simulink model "HydOilTemp_harness"  (Simulink 7.7)
settings: Solver=FixedStepDiscrete  SolverMode=SingleTasking  StartTime=0.0  StopTime=100  FixedStep=0.1  RelTol=1e-3
InitFcn:
  | CD_HOT_FILTER_GAIN.DataType = 'uint8';
  | CD_HOT_FILTER_GAIN.Value = 3;
  | 
  | if signalbuilder('HydOilTemp_harness/Signal_Builder','activegroup') == 3
  |   CD_SHUTDOWN_FUNCTION.DataType = 'uint8';
  |   CD_SHUTDOWN_FUNCTION.Value = 255;
  | elseif signalbuilder('HydOilTemp_harness/Signal_Builder','activegroup') == 6
  |   CD_SHUTDOWN_FUNCTION.DataType = 'uint8';
  |   CD_SHUTDOWN_FUNCTION.Value = 255;
  | else
  |  CD_SHUTDOWN_FUNCTION.DataType = 'uint8';
  |   CD_SHUTDOWN_FUNCTION.Value = 0;
  | end
  | 
  | if signalbuilder('HydOilTemp_harness/Signal_Builder','activegroup') == 1
  |   CD_HOT_FUNCTION.DataType = 'uint8';
  |   CD_HOT_FUNCTION.Value = 255;
  | elseif signalbuilder('HydOilTemp_harness/Signal_Builder','activegroup') == 5
  |   CD_HOT_FUNCTION.DataType = 'uint8';
  |   CD_HOT_FUNCTION.Value = 1;
  | elseif signalbuilder('HydOilTemp_harness/Signal_Builder','activegroup') == 6
  |   CD_HOT_FUNCTION.DataType = 'uint8';
  |   CD_HOT_FUNCTION.Value = 1;
  | else
  |   CD_HOT_FUNCTION.DataType = 'uint8';
  |   CD_HOT_FUNCTION.Value = 0;
  | end
undefined symbols (not defined in the file): CD_HOT_DEBOUNCE_EXTREMELY_HIGH, CD_HOT_DEBOUNCE_NORMAL, CD_HOT_DEBOUNCE_SHUTDOWN, CD_HOT_SWITCH_EXTREMELY_HIGH, EXTREMELY_HIGH, INIT_NORMAL, MXGTW_HOTGAUGE, MXGTW_HOTSND, NON_FUNCTIONAL, NORMAL, SENDER, SHUTDOWN, sigbuilder_block, srate100, SWITCH_INPUT, SYS_NORMAL
libraries: MX_Library x4, simulink x3
CloseFcn:
  | rtwprivate ssgencode ModelCloseRequest sle_main_controller
settings Model: Creator=smindema  LastModifiedBy=aliebel  RecordCoverage=on  CovMetricSettings=dcmtw  CovHTMLOptions=-aTS=1 -bRG=1 -bTC=1 -hTR=0 -nFC=0 -scm=1 -bcm=1 -xEv=0  CovCumulativeReport=on  CovModelRefEnable=off
settings MATStruct: SampleTime=0.01  Offset=0  Priority=[1.0]
settings DataIOCC: LimitDataPoints=off  SaveOutput=off  SaveTime=off
settings OptimizationCC: BlockReduction=off  InlineParams=on  ExpressionFolding=off  StateBitsets=on  DataBitsets=on  UseTempVars=on  InitFltsAndDblsToZero=on  NoFixptDivByZeroProtection=on  EfficientFloat2IntCast=on  OptimizeModelRefInitCode=on
settings DebuggingCC: SaveWithParameterizedLinksMsg=none  MultiTaskDSMMsg=warning  MultiTaskCondExecSysMsg=none  IntegerOverflowMsg=none  ModelReferenceCSMismatchMessage=warning
settings HardwareCC: ProdBitPerInt=16  ProdBitPerPointer=16  ProdIntDivRoundTo=Floor  ProdEndianess=BigEndian  ProdWordSize=16  ProdHWDeviceType=Motorola HC12
settings ModelReferenceCC: ModelReferenceNumInstancesAllowed=Single
settings RTWCC: SystemTargetFile=ert.tlc  GenCodeOnly=on  TemplateMakefile=ert_default_tmf  Description=Real-Time Workshop Embedded Coder (no auto configuration)  GenerateReport=on  RetainRTWFile=on  ProcessScript=ert_make_rtw_hook  IncludeHyperlinkInReport=on  LaunchReport=on  IncludeERTFirstTime=on
settings RTWCC: CustomHeaderCode=|
  | #include "cpp_req_defines.h"
  | #include "hw_fin.h"
  | #include "cdata.h"
settings CodeAppCC: IgnoreCustomStorageClasses=off  DefineNamingRule=UpperCase
settings ERTTargetCC: TargetFcnLib=ansi_tfl_tmw.mat  FunctionExecutionProfile=off  MultiwordLength=2048  GenerateSampleERTMain=on  IncludeMdlTerminateFcn=off  SupportAbsoluteTime=off  SupportNonFinite=off  SupportComplex=off  PurelyIntegerCode=on  ERTCustomFileTemplate=gen_rtw_req_defines_h.tlc  GlobalDataDefinition=InSeparateSourceFile  GlobalDataReference=InSeparateHeaderFile  ConvertIfToSwitch=off

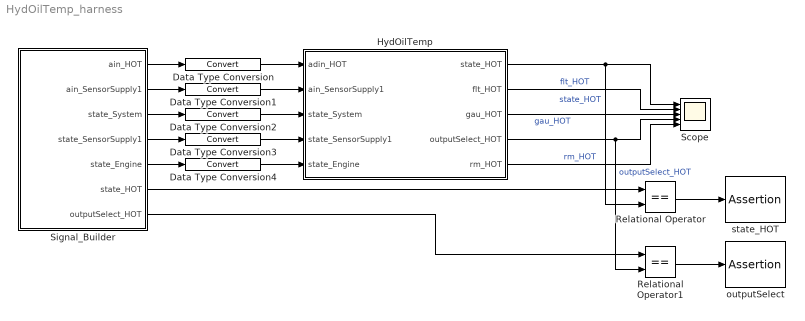
== system HydOilTemp_harness ==
  Data Type Conversion{,1..4} (5 alike) : DataTypeConversion
  HydOilTemp : Subsystem  TreatAsAtomicUnit=on  SystemSampleTime=srate100  RTWFileName=mod_Inputs
      settings: RTWSystemCode=Function  RTWFcnNameOpts=Use subsystem name  RTWFileNameOpts=User specified
  Relational Operator : RelationalOperator  Operator===  OutDataTypeStr=boolean
  Relational Operator1 : RelationalOperator  Operator===  OutDataTypeStr=boolean
  Scope : Scope  NumInputPorts=5
      settings: TimeRange=100  YMin=8~125~0~-1~550  YMax=15~350~17.5~1~950  MaxDataPoints=50000
  Signal_Builder : Subsystem  Tag=STV Subsys  LoadFcn=sigbuilder_block('load');  StartFcn=sigbuilder_block('start');  StopFcn=sigbuilder_block('stop');  ClipboardFcn=sigbuilder_block('clipboard');  mask(Sigbuilder block){}
      mask help: Sigbuilder GUI
      mask init:
      | if ~strcmp(get_param(bdroot(gcbh),'SimulationStatus'),'stopped') tuvar = sigbuilder_block('maskInit'); end
      settings: CopyFcn=sigbuilder_block('copy');  DeleteFcn=sigbuilder_block('delete');  ModelCloseFcn=sigbuilder_block('modelClose');  PreSaveFcn=sigbuilder_block('preSave');  NameChangeFcn=sigbuilder_block('namechange');  OpenFcn=sigbuilder_block('open',[348 297.75 957.75 420.75 ]);  CloseFcn=sigbuilder_block('close');
      mask Display: plot(0,0,100,100,[10,10,40,40,10],[80,20,20,80,80],[40,10],[50,50], [40,27,10],[65,72,56],[40,25,25,10],[28,28,43,43]);
  outputSelect : Assertion  Enabled=off
  state_HOT : Assertion  Enabled=off
  wires:
  Signal_Builder/1(ain_HOT) -> Data Type Conversion/1
  Signal_Builder/2(ain_SensorSupply1) -> Data Type Conversion1/1
  Data Type Conversion/1 -> HydOilTemp/1(adin_HOT)
  HydOilTemp/1(state_HOT) -> Scope/1, Relational Operator/2  "state_HOT"
  HydOilTemp/2(flt_HOT) -> Scope/2  "flt_HOT"
  HydOilTemp/3(gau_HOT) -> Scope/3  "gau_HOT"
  HydOilTemp/4(outputSelect_HOT) -> Scope/4, Relational Operator1/2  "outputSelect_HOT"
  HydOilTemp/5(rm_HOT) -> Scope/5  "rm_HOT"
  Data Type Conversion1/1 -> HydOilTemp/2(ain_SensorSupply1)
  Data Type Conversion2/1 -> HydOilTemp/3(state_System)
  Data Type Conversion3/1 -> HydOilTemp/4(state_SensorSupply1)
  Data Type Conversion4/1 -> HydOilTemp/5(state_Engine)
  Signal_Builder/3(state_System) -> Data Type Conversion2/1
  Signal_Builder/4(state_SensorSupply1) -> Data Type Conversion3/1
  Signal_Builder/5(state_Engine) -> Data Type Conversion4/1
  Relational Operator/1 -> state_HOT/1
  Relational Operator1/1 -> outputSelect/1
  Signal_Builder/6(state_HOT) -> Relational Operator/1
  Signal_Builder/7(outputSelect_HOT) -> Relational Operator1/1

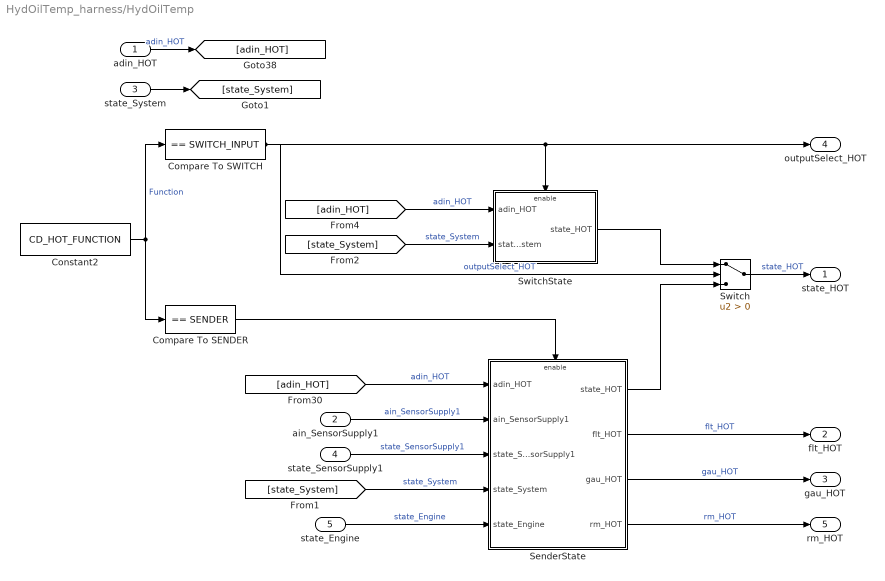
== system HydOilTemp_harness/HydOilTemp ==
  adin_HOT : Inport  OutDataTypeStr=uint16
  ain_SensorSupply1 : Inport  Port=2  OutDataTypeStr=uint16
  state_System : Inport  Port=3
  state_SensorSupply1 : Inport  Port=4  OutDataTypeStr=uint8
  state_Engine : Inport  Port=5  OutDataTypeStr=uint8
  Compare To SENDER : simulink/Logic and Bit Operations/Compare To Constant  SystemSampleTime=-1  relop===  const=SENDER  LogicOutDataTypeMode=boolean  ZeroCross=off
  Compare To SWITCH : simulink/Logic and Bit Operations/Compare To Constant  SystemSampleTime=-1  relop===  const=SWITCH_INPUT  LogicOutDataTypeMode=boolean  ZeroCross=off
  Constant2 : Constant  Value=CD_HOT_FUNCTION  OutDataTypeStr=uint8
  SenderState : Subsystem  TreatAsAtomicUnit=on
  Switch : Switch  Criteria=u2 > Threshold  ZeroCross=off
      settings: AttributesFormatString=<threshold=%<Threshold>>
  SwitchState : Subsystem  TreatAsAtomicUnit=on
  state_HOT : Outport  OutDataTypeStr=uint8
  flt_HOT : Outport  Port=2  OutDataTypeStr=uint16
  gau_HOT : Outport  Port=3  OutDataTypeStr=uint16
  outputSelect_HOT : Outport  Port=4
  rm_HOT : Outport  Port=5  OutDataTypeStr=uint16
  wires:
  state_SensorSupply1/1 -> SenderState/3(state_SensorSupply1)  "state_SensorSupply1"
  ain_SensorSupply1/1 -> SenderState/2(ain_SensorSupply1)  "ain_SensorSupply1"
  [adin_HOT] -> SenderState/1(adin_HOT)  "adin_HOT"
  [adin_HOT] -> SwitchState/1(adin_HOT)  "adin_HOT"
  Switch/1 -> state_HOT/1  "state_HOT"
  SwitchState/1(state_HOT) -> Switch/1
  SenderState/1(state_HOT) -> Switch/3
  SenderState/3(gau_HOT) -> gau_HOT/1  "gau_HOT"
  SenderState/2(flt_HOT) -> flt_HOT/1  "flt_HOT"
  adin_HOT/1 -> [adin_HOT]  "adin_HOT"
  Constant2/1 -> Compare To SWITCH/1, Compare To SENDER/1  "Function"
  Compare To SENDER/1 -> SenderState/Enable
  Compare To SWITCH/1 -> Switch/2, SwitchState/Enable, outputSelect_HOT/1  "outputSelect_HOT"
  [state_System] -> SenderState/4(state_System)  "state_System"
  state_System/1 -> [state_System]
  [state_System] -> SwitchState/2(state_System)  "state_System"
  SenderState/4(rm_HOT) -> rm_HOT/1  "rm_HOT"
  state_Engine/1 -> SenderState/5(state_Engine)  "state_Engine"

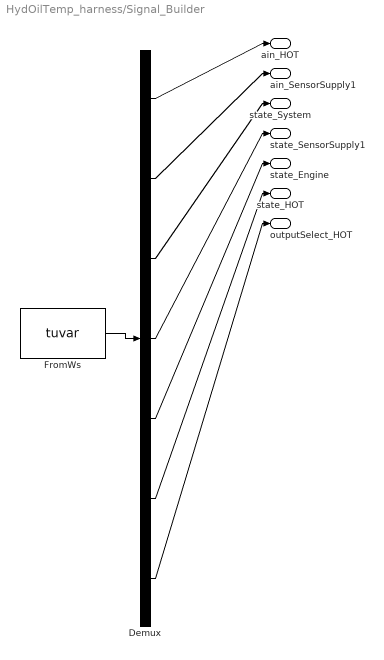
== system HydOilTemp_harness/Signal_Builder ==
  Demux : Demux  Tag=STV Demux  Outputs=7
  FromWs : FromWorkspace  Tag=STV FromWs  VariableName=tuvar  SampleTime=0  SigBuilderData=DataTag0  VnvData=DataTag1
      SigBuilderData=|
      | common.afterFinalStr = 'Extrapolate'
      | common.sampleTime = 0
      | dataSet(1).timeRange = [0 100]
      | dataSet(1).name = 'T1-Nonfunc'
      | dataSet(2).timeRange = [0 100]
      | dataSet(2).name = 'T2-OOR'
      | dataSet(3).timeRange = [0 100]
      | dataSet(3).name = 'T3-HIGH'
      | dataSet(4).timeRange = [0 100]
      | dataSet(4).name = 'T4-EXTHIGH'
      | dataSet(5).timeRange = [0 100]
      | dataSet(5).name = 'T5-SWITCH'
      | dataSet(6).timeRange = [0 100]
      | dataSet(6).name = 'T6-SWITCH no shut'
      | dataSet(7).timeRange = [0 100]
      | dataSet(7).name = 'TABLE'
      | dataSet(8).timeRange = [0 100]
      | dataSet(8).name = 'TABLE1'
      | sbobj.Groups(1).Name = 'T1-Nonfunc'
      | sbobj.Groups(1).Signals(1).Name = 'ain_HOT'
      | sbobj.Groups(1).Signals(1).XData = [0 100]
      | sbobj.Groups(1).Signals(1).YData = [380 380]
      | sbobj.Groups(1).Signals(2).Name = 'ain_SensorSupply1'
      | sbobj.Groups(1).Signals(2).XData = [0 100]
      | sbobj.Groups(1).Signals(2).YData = [850 850]
      | sbobj.Groups(1).Signals(3).Name = 'state_System'
      | sbobj.Groups(1).Signals(3).XData = [0 0.6 0.6 100]
      | sbobj.Groups(1).Signals(3).YData = [0 0 1 1]
      | sbobj.Groups(1).Signals(4).Name = 'state_SensorSupply1'
      | sbobj.Groups(1).Signals(4).XData = [0 100]
      | sbobj.Groups(1).Signals(4).YData = [8 8]
      | sbobj.Groups(1).Signals(5).Name = 'state_Engine'
      | sbobj.Groups(1).Signals(5).XData = [0 100]
      | sbobj.Groups(1).Signals(5).YData = [3 3]
      | sbobj.Groups(1).Signals(6).Name = 'state_HOT'
      | sbobj.Groups(1).Signals(6).XData = [0 100]
      | sbobj.Groups(1).Signals(6).YData = [8 8]
      | sbobj.Groups(1).Signals(7).Name = 'outputSelect_HOT'
      | sbobj.Groups(1).Signals(7).XData = [0 100]
      | sbobj.Groups(1).Signals(7).YData = [0 0]
      | sbobj.Groups(2).Name = 'T2-OOR'
      | sbobj.Groups(2).Signals(1).Name = 'ain_HOT'
      | sbobj.Groups(2).Signals(1).XData = [0 0.4 0.4 0.9 0.9 34.6 34.6 35 35 36.3 36.3 38.4 38.4 39.7 39.7 40.4 40.4 75 75 75.4 75.4 76.3 76.3 100]
      | sbobj.Groups(2).Signals(1).YData = [0 0 600 600 0 0 280 290 0 0 500 500 1020 1010 420 430 1020 1020 230 240 1000 998.269230769 640 640]
      | sbobj.Groups(2).Signals(2).Name = 'ain_SensorSupply1'
      | sbobj.Groups(2).Signals(2).XData = [0 100]
      | sbobj.Groups(2).Signals(2).YData = [850 850]
      | sbobj.Groups(2).Signals(3).Name = 'state_System'
      | sbobj.Groups(2).Signals(3).XData = [0 0.2 0.2 100]
      | sbobj.Groups(2).Signals(3).YData = [0 0 1 1]
      | sbobj.Groups(2).Signals(4).Name = 'state_SensorSupply1'
      | sbobj.Groups(2).Signals(4).XData = [0 2.7 2.7 3.1 3.1 33.6 33.6 33.8 33.8 41.8 41.8 42.4 42.4 73.1 73.1 73.8 73.8 100]
      | sbobj.Groups(2).Signals(4).YData = [8 8 6.98 6.98 8 8 6.98 6.98 8 8 7 7 8 8 7 7 8 8]
      | sbobj.Groups(2).Signals(5).Name = 'state_Engine'
      | sbobj.Groups(2).Signals(5).XData = [0 100]
      | sbobj.Groups(2).Signals(5).YData = [0 0]
      | sbobj.Groups(2).Signals(6).Name = 'state_HOT'
      | sbobj.Groups(2).Signals(6).XData = [0 33.3 33.3 41.8 41.8 72.6 72.6 81.4 81.4 100]
      | sbobj.Groups(2).Signals(6).YData = [8 8 22 22 8 8 21 21 8 8]
      | sbobj.Groups(2).Signals(7).Name = 'outputSelect_HOT'
      | sbobj.Groups(2).Signals(7).XData = [0 100]
      | sbobj.Groups(2).Signals(7).YData = [0 0]
      | sbobj.Groups(3).Name = 'T3-HIGH'
      | sbobj.Groups(3).Signals(1).Name = 'ain_HOT'
      | sbobj.Groups(3).Signals(1).XData = [0 2.2 2.2 7 7 7.5 7.5 18.2 18.2 18.5 18.5 29.7 29.7 30.8 30.8 31.7 31.7 39 39 39.5 39.5 50.1 50.1 55.4 55.4 63.6 63.6 64.1 64.1 70.1 70.1 76.4 76.4 77.6 77.6 83.8 83.8 94.8 94.8 97.8 97.8 100]
      | sbobj.Groups(3).Signals(1).YData = [500 500 695 695 500 495 695 695 500 500 695 695 455 450 600 600 455 455 600 600 455 455 700 700 780 780 635 635 780 780 700 700 600 600 700 700 590 590 770 770 590 590]
      | sbobj.Groups(3).Signals(2).Name = 'ain_SensorSupply1'
      | sbobj.Groups(3).Signals(2).XData = [0 100]
      | sbobj.Groups(3).Signals(2).YData = [850 850]
      | sbobj.Groups(3).Signals(3).Name = 'state_System'
      | sbobj.Groups(3).Signals(3).XData = [0 100]
      | sbobj.Groups(3).Signals(3).YData = [1 1]
      | sbobj.Groups(3).Signals(4).Name = 'state_SensorSupply1'
      | sbobj.Groups(3).Signals(4).XData = [0 100]
      | sbobj.Groups(3).Signals(4).YData = [8 8]
      | sbobj.Groups(3).Signals(5).Name = 'state_Engine'
      | sbobj.Groups(3).Signals(5).XData = [0 3.7 3.7 22.8 22.8 24.3 24.3 41.7 41.7 42.3 42.3 67 67 67.9 67.9 100]
      | sbobj.Groups(3).Signals(5).YData = [0 0 3 3 1 1 3 3 1 1 3 3 0.95 0.95 3 3]
      | sbobj.Groups(3).Signals(6).Name = 'state_HOT'
      | sbobj.Groups(3).Signals(6).XData = [0 14.7 14.7 37 37 63.4 63.4 89 89 100]
      | sbobj.Groups(3).Signals(6).YData = [8 8 10 10 12 12 11 11 8 8]
      | sbobj.Groups(3).Signals(7).Name = 'outputSelect_HOT'
      | sbobj.Groups(3).Signals(7).XData = [0 100]
      | sbobj.Groups(3).Signals(7).YData = [0 0]
      | sbobj.Groups(4).Name = 'T4-EXTHIGH'
      | sbobj.Groups(4).Signals(1).Name = 'ain_HOT'
      | sbobj.Groups(4).Signals(1).XData = [0 1 1 8.9 8.9 21 21 21.4 21.4 58.4 58.4 76.4 76.4 77.6 77.6 83.8 83.8 94.8 94.8 97.8 97.8 100]
      | sbobj.Groups(4).Signals(1).YData = [1040 1040 700 700 770 770 400 400 770 780 700 700 600 600 700 700 590 590 770 770 590 590]
      | sbobj.Groups(4).Signals(2).Name = 'ain_SensorSupply1'
      | sbobj.Groups(4).Signals(2).XData = [0 87.2 100]
      | sbobj.Groups(4).Signals(2).YData = [850 850 850]
      | sbobj.Groups(4).Signals(3).Name = 'state_System'
      | sbobj.Groups(4).Signals(3).XData = [0 0.7 0.7 91.9 91.9 93 93 100]
      | sbobj.Groups(4).Signals(3).YData = [0 0 1 1 0 0 1 1]
      | sbobj.Groups(4).Signals(4).Name = 'state_SensorSupply1'
      | sbobj.Groups(4).Signals(4).XData = [0 85 85 87 87 100]
      | sbobj.Groups(4).Signals(4).YData = [8 8 7 7 8 8]
      | sbobj.Groups(4).Signals(5).Name = 'state_Engine'
      | sbobj.Groups(4).Signals(5).XData = [0 32 32 33.7 33.7 100]
      | sbobj.Groups(4).Signals(5).YData = [3 3 2 2 3 3]
      | sbobj.Groups(4).Signals(6).Name = 'state_HOT'
      | sbobj.Groups(4).Signals(6).XData = [0 15 15 54 54 85 85 100]
      | sbobj.Groups(4).Signals(6).YData = [8 8 11 11 15 15 8 8]
      | sbobj.Groups(4).Signals(7).Name = 'outputSelect_HOT'
      | sbobj.Groups(4).Signals(7).XData = [0 100]
      | sbobj.Groups(4).Signals(7).YData = [0 0]
      | sbobj.Groups(5).Name = 'T5-SWITCH'
      | sbobj.Groups(5).Signals(1).Name = 'ain_HOT'
      | sbobj.Groups(5).Signals(1).XData = [0 9.8 9.8 13 13 18 18 20 20 22 22 34 34 35.4 35.4 50 50 60.8 60.8 97.8 97.8 100]
      | sbobj.Groups(5).Signals(1).YData = [1024 1024 0 0 1024 1024 0 0 1000 1000 0 0 980 980 0 0 1024 1024 0 0 1040 1040]
      | sbobj.Groups(5).Signals(2).Name = 'ain_SensorSupply1'
      | sbobj.Groups(5).Signals(2).XData = [0 100]
      | sbobj.Groups(5).Signals(2).YData = [850 850]
      | sbobj.Groups(5).Signals(3).Name = 'state_System'
      | sbobj.Groups(5).Signals(3).XData = [0 8.6 8.6 11.5 11.5 100]
      | sbobj.Groups(5).Signals(3).YData = [1 1 0 0 1 1]
      | sbobj.Groups(5).Signals(4).Name = 'state_SensorSupply1'
      | sbobj.Groups(5).Signals(4).XData = [0 100]
      | sbobj.Groups(5).Signals(4).YData = [8 8]
      | sbobj.Groups(5).Signals(5).Name = 'state_Engine'
      | sbobj.Groups(5).Signals(5).XData = [0 100]
      | sbobj.Groups(5).Signals(5).YData = [0 0]
      | sbobj.Groups(5).Signals(6).Name = 'state_HOT'
      | sbobj.Groups(5).Signals(6).XData = [0 32.1 32.1 55.2 55.2 70.9 70.9 91.1 91.1 100]
      | sbobj.Groups(5).Signals(6).YData = [8 8 11 11 8 8 11 11 15 15]
      | sbobj.Groups(5).Signals(7).Name = 'outputSelect_HOT'
      | sbobj.Groups(5).Signals(7).XData = [0 100]
      | sbobj.Groups(5).Signals(7).YData = [1 1]
      | sbobj.Groups(6).Name = 'T6-SWITCH no shut'
      | sbobj.Groups(6).Signals(1).Name = 'ain_HOT'
      | sbobj.Groups(6).Signals(1).XData = [0 9.8 9.8 13 13 18 18 20 20 22 22 42.6 42.6 44.8 44.8 50 50 60.8 60.8 79.4 79.4 100]
      | sbobj.Groups(6).Signals(1).YData = [1024 1024 0 0 1024 1024 0 0 1000 1000 0 0 980 980 0 0 1024 1024 0 0 1040 1040]
      | sbobj.Groups(6).Signals(2).Name = 'ain_SensorSupply1'
      | sbobj.Groups(6).Signals(2).XData = [0 100]
      | sbobj.Groups(6).Signals(2).YData = [850 850]
      | sbobj.Groups(6).Signals(3).Name = 'state_System'
      | sbobj.Groups(6).Signals(3).XData = [0 8.6 8.6 11.5 11.5 28.2 28.2 31 31 72.1 72.1 82.8 82.8 100]
      | sbobj.Groups(6).Signals(3).YData = [1 1 0 0 1 1 0 0 1 1 0 0 1 1]
      | sbobj.Groups(6).Signals(4).Name = 'state_SensorSupply1'
      | sbobj.Groups(6).Signals(4).XData = [0 100]
      | sbobj.Groups(6).Signals(4).YData = [8 8]
      | sbobj.Groups(6).Signals(5).Name = 'state_Engine'
      | sbobj.Groups(6).Signals(5).XData = [0 100]
      | sbobj.Groups(6).Signals(5).YData = [0 0]
      | sbobj.Groups(6).Signals(6).Name = 'state_HOT'
      | sbobj.Groups(6).Signals(6).XData = [0 41.1 41.1 55.1 55.1 70.9 70.9 77.2 77.2 100]
      | sbobj.Groups(6).Signals(6).YData = [8 8 11 11 8 8 11 11 8 8]
      | sbobj.Groups(6).Signals(7).Name = 'outputSelect_HOT'
      | sbobj.Groups(6).Signals(7).XData = [0 100]
      | sbobj.Groups(6).Signals(7).YData = [1 1]
      | sbobj.Groups(7).Name = 'TABLE'
      | sbobj.Groups(7).Signals(1).Name = 'ain_HOT'
      | sbobj.Groups(7).Signals(1).XData = [0 100]
      | sbobj.Groups(7).Signals(1).YData = [500 1024]
      | sbobj.Groups(7).Signals(2).Name = 'ain_SensorSupply1'
      | sbobj.Groups(7).Signals(2).XData = [0 100]
      | sbobj.Groups(7).Signals(2).YData = [850 850]
      | sbobj.Groups(7).Signals(3).Name = 'state_System'
      | sbobj.Groups(7).Signals(3).XData = [0 0.6 0.6 100]
      | sbobj.Groups(7).Signals(3).YData = [0 0 1 1]
      | sbobj.Groups(7).Signals(4).Name = 'state_SensorSupply1'
      | sbobj.Groups(7).Signals(4).XData = [0 100]
      | sbobj.Groups(7).Signals(4).YData = [8 8]
      | sbobj.Groups(7).Signals(5).Name = 'state_Engine'
      | sbobj.Groups(7).Signals(5).XData = [0 100]
      | sbobj.Groups(7).Signals(5).YData = [3 3]
      | sbobj.Groups(7).Signals(6).Name = 'state_HOT'
      | sbobj.Groups(7).Signals(6).XData = [0 5.8 5.8 15.6 15.6 48.4 48.4 84.8 84.8 100]
      | sbobj.Groups(7).Signals(6).YData = [8 8 12 12 8 8 11 11 21 21]
      | sbobj.Groups(7).Signals(7).Name = 'outputSelect_HOT'
      | sbobj.Groups(7).Signals(7).XData = [0 100]
      | sbobj.Groups(7).Signals(7).YData = [0 0]
      | sbobj.Groups(8).Name = 'TABLE1'
      | sbobj.Groups(8).Signals(1).Name = 'ain_HOT'
      | sbobj.Groups(8).Signals(1).XData = [0 100]
      | sbobj.Groups(8).Signals(1).YData = [500 0]
      | sbobj.Groups(8).Signals(2).Name = 'ain_SensorSupply1'
      | sbobj.Groups(8).Signals(2).XData = [0 100]
      | sbobj.Groups(8).Signals(2).YData = [850 850]
      | sbobj.Groups(8).Signals(3).Name = 'state_System'
      | sbobj.Groups(8).Signals(3).XData = [0 0.6 0.6 100]
      | sbobj.Groups(8).Signals(3).YData = [0 0 1 1]
      | sbobj.Groups(8).Signals(4).Name = 'state_SensorSupply1'
      | sbobj.Groups(8).Signals(4).XData = [0 100]
      | sbobj.Groups(8).Signals(4).YData = [8 8]
      | sbobj.Groups(8).Signals(5).Name = 'state_Engine'
      | sbobj.Groups(8).Signals(5).XData = [0 100]
      | sbobj.Groups(8).Signals(5).YData = [3 3]
      | sbobj.Groups(8).Signals(6).Name = 'state_HOT'
      | sbobj.Groups(8).Signals(6).XData = [0 5.8 5.8 100]
      | sbobj.Groups(8).Signals(6).YData = [8 8 12 12]
      | sbobj.Groups(8).Signals(7).Name = 'outputSelect_HOT'
      | sbobj.Groups(8).Signals(7).XData = [0 100]
      | sbobj.Groups(8).Signals(7).YData = [0 0]
  ain_HOT : Outport  Tag=STV Outport
  ain_SensorSupply1 : Outport  Tag=STV Outport  Port=2
  state_System : Outport  Tag=STV Outport  Port=3
  state_SensorSupply1 : Outport  Tag=STV Outport  Port=4
  state_Engine : Outport  Tag=STV Outport  Port=5
  state_HOT : Outport  Tag=STV Outport  Port=6
  outputSelect_HOT : Outport  Tag=STV Outport  Port=7
  wires:
  FromWs/1 -> Demux/1
  Demux/1 -> ain_HOT/1
  Demux/2 -> ain_SensorSupply1/1
  Demux/3 -> state_System/1
  Demux/4 -> state_SensorSupply1/1
  Demux/5 -> state_Engine/1
  Demux/6 -> state_HOT/1
  Demux/7 -> outputSelect_HOT/1

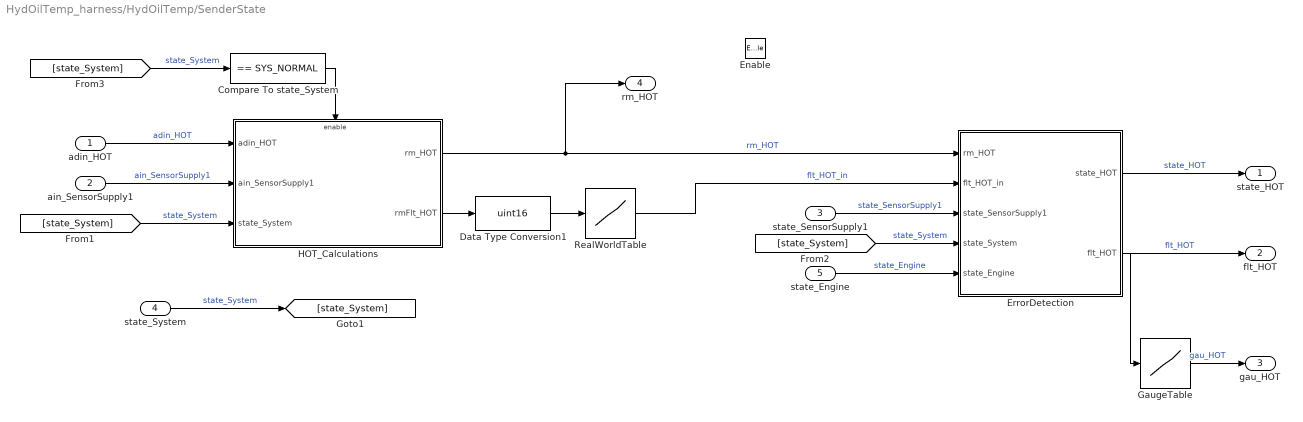
== system HydOilTemp_harness/HydOilTemp/SenderState ==
  adin_HOT : Inport  OutDataTypeStr=uint16
  ain_SensorSupply1 : Inport  Port=2  OutDataTypeStr=uint16
  state_SensorSupply1 : Inport  Port=3  OutDataTypeStr=uint8
  state_System : Inport  Port=4
  state_Engine : Inport  Port=5
  Enable : EnablePort  PropagateVarSize=During execution
      settings: AttributesFormatString=<state=%<StatesWhenEnabling>>
  Compare To state_System : simulink/Logic and Bit Operations/Compare To Constant  SystemSampleTime=-1  relop===  const=SYS_NORMAL  LogicOutDataTypeMode=boolean  ZeroCross=off
  Data Type Conversion1 : DataTypeConversion  OutDataTypeStr=uint16
  ErrorDetection : Stateflow chart  TreatAsAtomicUnit=on
  GaugeTable : Lookup  InputValues=[0:340]  Table=MXGTW_HOTGAUGE  LookUpMeth=Use Input Nearest  OutDataTypeStr=uint16  RndMeth=Zero  SaturateOnIntegerOverflow=on
      settings: AttributesFormatString=input = %<InputValues>\noutput = %<OutputValues>\nlookup = %<LookUpMeth>\nrounding = %<RndMeth>
  HOT_Calculations : Subsystem
  RealWorldTable : Lookup  InputValues=MXGTW_HOTSND  Table=[0:340]  LookUpMeth=Use Input Nearest  OutDataTypeStr=uint16  RndMeth=Zero  SaturateOnIntegerOverflow=on
      settings: AttributesFormatString=input = %<InputValues>\noutput = %<OutputValues>\nlookup = %<LookUpMeth>\nrounding = %<RndMeth>
  state_HOT : Outport  InitialOutput=[INIT_NORMAL]
  flt_HOT : Outport  Port=2  InitialOutput=[0]
  gau_HOT : Outport  Port=3  InitialOutput=[0]
  rm_HOT : Outport  Port=4  InitialOutput=[0]
  wires:
  state_SensorSupply1/1 -> ErrorDetection/3(state_SensorSupply1)  "state_SensorSupply1"
  ErrorDetection/1(state_HOT) -> state_HOT/1  "state_HOT"
  GaugeTable/1 -> gau_HOT/1  "gau_HOT"
  RealWorldTable/1 -> ErrorDetection/2(flt_HOT_in)  "flt_HOT_in"
  ain_SensorSupply1/1 -> HOT_Calculations/2(ain_SensorSupply1)  "ain_SensorSupply1"
  adin_HOT/1 -> HOT_Calculations/1(adin_HOT)  "adin_HOT"
  HOT_Calculations/2(rmFlt_HOT) -> Data Type Conversion1/1
  [state_System] -> ErrorDetection/4(state_System)  "state_System"
  state_Engine/1 -> ErrorDetection/5(state_Engine)  "state_Engine"
  ErrorDetection/2(flt_HOT) -> flt_HOT/1, GaugeTable/1  "flt_HOT"
  state_System/1 -> [state_System]  "state_System"
  HOT_Calculations/1(rm_HOT) -> ErrorDetection/1(rm_HOT), rm_HOT/1  "rm_HOT"
  [state_System] -> HOT_Calculations/3(state_System)  "state_System"
  Data Type Conversion1/1 -> RealWorldTable/1
  Compare To state_System/1 -> HOT_Calculations/Enable
  [state_System] -> Compare To state_System/1  "state_System"

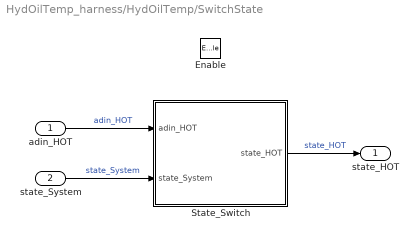
== system HydOilTemp_harness/HydOilTemp/SwitchState ==
  adin_HOT : Inport
  state_System : Inport  Port=2
  Enable : EnablePort  PropagateVarSize=During execution
      settings: AttributesFormatString=<state=%<StatesWhenEnabling>>
  State_Switch : Stateflow chart  TreatAsAtomicUnit=on
  state_HOT : Outport  InitialOutput=[INIT_NORMAL]
  wires:
  State_Switch/1(state_HOT) -> state_HOT/1  "state_HOT"
  adin_HOT/1 -> State_Switch/1(adin_HOT)  "adin_HOT"
  state_System/1 -> State_Switch/2(state_System)  "state_System"

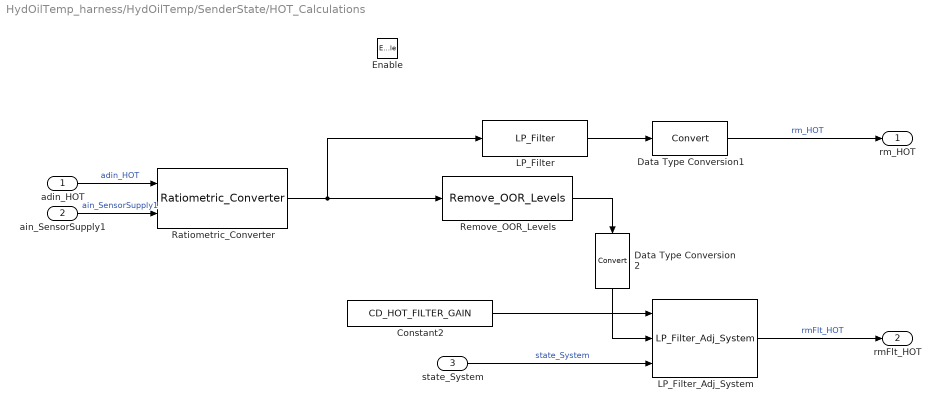
== system HydOilTemp_harness/HydOilTemp/SenderState/HOT_Calculations ==
  adin_HOT : Inport  OutDataTypeStr=uint16
  ain_SensorSupply1 : Inport  Port=2  OutDataTypeStr=uint16
  state_System : Inport  Port=3  OutDataTypeStr=uint8
  Enable : EnablePort  StatesWhenEnabling=reset  PropagateVarSize=During execution
  Constant2 : Constant  Value=CD_HOT_FILTER_GAIN  OutDataTypeStr=uint8
  Data Type Conversion1 : DataTypeConversion
  Data Type Conversion2 : DataTypeConversion
  LP_Filter : MX_Library/LP_Filter  SystemSampleTime=-1  GAIN=3
  LP_Filter_Adj_System : MX_Library/LP_Filter_Adj_System  SystemSampleTime=-1
  Ratiometric_Converter : MX_Library/Ratiometric_Converter  SystemSampleTime=-1  multiplier=1000
  Remove_OOR_Levels : MX_Library/Remove_OOR_Levels  SystemSampleTime=-1  OORL_LEVEL=CD_HOT_OORL  OORH_LEVEL=CD_HOT_OORH
  rm_HOT : Outport  InitialOutput=[0]
  rmFlt_HOT : Outport  Port=2  InitialOutput=[0]
  wires:
  Remove_OOR_Levels/1 -> Data Type Conversion2/1
  Data Type Conversion1/1 -> rm_HOT/1  "rm_HOT"
  Ratiometric_Converter/1 -> Remove_OOR_Levels/1, LP_Filter/1
  ain_SensorSupply1/1 -> Ratiometric_Converter/2  "ain_SensorSupply1"
  adin_HOT/1 -> Ratiometric_Converter/1  "adin_HOT"
  LP_Filter_Adj_System/1 -> rmFlt_HOT/1  "rmFlt_HOT"
  Data Type Conversion2/1 -> LP_Filter_Adj_System/2
  LP_Filter/1 -> Data Type Conversion1/1
  Constant2/1 -> LP_Filter_Adj_System/1
  state_System/1 -> LP_Filter_Adj_System/3  "state_System"

== stateflow chart HydOilTemp/SwitchState/State_Switch ==
  state NORMAL
    state NORMAL
      en:state_HOT = NORMAL;
    state DEBOUNCE
      en:debounceCount = 0;
      du:debounceCount++;
    (default) -> NORMAL.DEBOUNCE
    NORMAL.DEBOUNCE -> NORMAL.NORMAL : [(debounceCount >= CD_HOT_DEBOUNCE_NORMAL)...
        | || (state_HOT == NORMAL)]
  state SHUTDOWN
    state DEBOUNCE
      en:debounceCount = 0;
      du:debounceCount++;
    state SHUTDOWN
      en:state_HOT = SHUTDOWN;
    (default) -> SHUTDOWN.DEBOUNCE
    SHUTDOWN.DEBOUNCE -> SHUTDOWN.SHUTDOWN : [(debounceCount >= CD_HOT_DEBOUNCE_SHUTDOWN)]
  state EXTREMELY_HIGH
    state EXTREMELY_HIGH
      en:state_HOT = EXTREMELY_HIGH;
    state DEBOUNCE
      en:debounceCount = 0;
      du:debounceCount++;
    EXTREMELY_HIGH.DEBOUNCE -> EXTREMELY_HIGH.EXTREMELY_HIGH : [(debounceCount >= CD_HOT_DEBOUNCE_EXTREMELY_HIGH)...
        | || (state_HOT== EXTREMELY_HIGH)]
    (default) -> EXTREMELY_HIGH.DEBOUNCE
  NORMAL -> EXTREMELY_HIGH : [(adin_HOT <= CD_HOT_SWITCH_EXTREMELY_HIGH)...
      | && (state_System == SYS_NORMAL)]
  SHUTDOWN -> EXTREMELY_HIGH : [(adin_HOT > CD_HOT_SWITCH_EXTREMELY_HIGH)...
      | && (state_HOT != SHUTDOWN)]
  EXTREMELY_HIGH -> NORMAL [order 1] : [(adin_HOT > CD_HOT_SWITCH_EXTREMELY_HIGH)...
      | || (state_System != SYS_NORMAL)]
  EXTREMELY_HIGH -> SHUTDOWN [order 2] : [(CD_SHUTDOWN_FUNCTION != NON_FUNCTIONAL)...
      | && (state_HOT == EXTREMELY_HIGH)]
  (default) -> NORMAL.NORMAL
  data: adin_HOT input uint16; state_HOT output uint8; debounceCount local uint16 =0; CD_HOT_DEBOUNCE_EXTREMELY_HIGH parameter uint16; CD_HOT_DEBOUNCE_NORMAL parameter uint16; CD_HOT_DEBOUNCE_SHUTDOWN parameter uint16; CD_SHUTDOWN_FUNCTION parameter uint8; EXTREMELY_HIGH parameter uint8 =10; NON_FUNCTIONAL parameter uint8 =255; SHUTDOWN parameter uint8 =15; NORMAL parameter uint8 =8; state_System input uint8; SYS_NORMAL parameter uint8; CD_HOT_SWITCH_EXTREMELY_HIGH parameter uint16

== stateflow chart HydOilTemp/SenderState/ErrorDetection ==
  state ERROR_STATE [parallel]
    settings: executionOrder=2
    state NON_FUNCTIONAL
      en:state_HOT = NORMAL;
    state OORH
      state DEBOUNCE
        en:debounceCount = 0;
        du:debounceCount++;
      state NORMAL
        en:state_HOT = OORH;
      (default) -> ERROR_STATE.OORH.DEBOUNCE
      ERROR_STATE.OORH.DEBOUNCE -> ERROR_STATE.OORH.NORMAL : [(debounceCount >= CD_HOT_DEBOUNCE_OORH)...
          | || (state_HOT == OORH)]
    state NORMAL
      state SHUTDOWN
        state DEBOUNCE
          en:debounceCount = 0;
          du:debounceCount++;
        state SHUTDOWN
          en:state_HOT = SHUTDOWN;
        (default) -> ERROR_STATE.NORMAL.SHUTDOWN.DEBOUNCE
        ERROR_STATE.NORMAL.SHUTDOWN.DEBOUNCE -> ERROR_STATE.NORMAL.SHUTDOWN.SHUTDOWN : [(debounceCount >= CD_HOT_DEBOUNCE_SHUTDOWN)]
      state EXTREMELY_HIGH
        state DEBOUNCE
          en:debounceCount = 0;
          du:debounceCount++;
        state NORMAL
          en:state_HOT = EXTREMELY_HIGH;
        (default) -> ERROR_STATE.NORMAL.EXTREMELY_HIGH.DEBOUNCE
        ERROR_STATE.NORMAL.EXTREMELY_HIGH.DEBOUNCE -> ERROR_STATE.NORMAL.EXTREMELY_HIGH.NORMAL : [(debounceCount >= CD_HOT_DEBOUNCE_EXTREMELY_HIGH)...
            | || (state_HOT == EXTREMELY_HIGH)]
      state HIGH
        state DEBOUNCE
          en:debounceCount = 0;
          du:debounceCount++;
        state HIGH
          en:state_HOT = HIGH;
        (default) -> ERROR_STATE.NORMAL.HIGH.DEBOUNCE
        ERROR_STATE.NORMAL.HIGH.DEBOUNCE -> ERROR_STATE.NORMAL.HIGH.HIGH : [(debounceCount >= CD_HOT_DEBOUNCE_HIGH)...
            | || (state_HOT == HIGH)]
      state NORMAL
        state DEBOUNCE
          en:debounceCount = 0;
          du:debounceCount++;
        state NORMAL
          en:state_HOT = NORMAL;
        (default) -> ERROR_STATE.NORMAL.NORMAL.DEBOUNCE
        ERROR_STATE.NORMAL.NORMAL.DEBOUNCE -> ERROR_STATE.NORMAL.NORMAL.NORMAL : [(debounceCount >= CD_HOT_DEBOUNCE_NORMAL)...
            | || (state_HOT == NORMAL)]
      state COLD
        state DEBOUNCE
          en:debounceCount = 0;
          du:debounceCount++;
        state COLD
          en:state_HOT = COLD;
        (default) -> ERROR_STATE.NORMAL.COLD.DEBOUNCE
        ERROR_STATE.NORMAL.COLD.DEBOUNCE -> ERROR_STATE.NORMAL.COLD.COLD : [(debounceCount >= CD_HOT_DEBOUNCE_COLD)...
            | || (state_HOT == COLD)]
      EXTREMELY_HIGH -> ERROR_STATE.NORMAL.SHUTDOWN [order 2] : [(CD_SHUTDOWN_FUNCTION != NON_FUNCTIONAL)...
          | && (state_HOT == EXTREMELY_HIGH)]
      ERROR_STATE.NORMAL.SHUTDOWN -> EXTREMELY_HIGH : [((flt_HOT < (CD_HOT_EXTREMELY_HIGH - CD_TEMPERATURE_HYSTERESIS)) || (state_Engine != ENGINE_RUNNING))...
          | && (state_HOT != SHUTDOWN)]
      ERROR_STATE.NORMAL.HIGH -> EXTREMELY_HIGH [order 2] : [(flt_HOT >= CD_HOT_EXTREMELY_HIGH)]
      EXTREMELY_HIGH -> ERROR_STATE.NORMAL.HIGH [order 1] : [(flt_HOT < (CD_HOT_EXTREMELY_HIGH - CD_TEMPERATURE_HYSTERESIS))...
          | || (state_Engine != ENGINE_RUNNING)]
      ERROR_STATE.NORMAL.HIGH -> ERROR_STATE.NORMAL.NORMAL [order 1] : [(flt_HOT < (CD_HOT_HIGH - CD_TEMPERATURE_HYSTERESIS))...
          | || (state_Engine != ENGINE_RUNNING)]
      ERROR_STATE.NORMAL.NORMAL -> ERROR_STATE.NORMAL.HIGH [order 2] : [(flt_HOT >= CD_HOT_HIGH)...
          | && (state_Engine == ENGINE_RUNNING)]
      (default) -> ERROR_STATE.NORMAL.NORMAL
      ERROR_STATE.NORMAL.NORMAL -> ERROR_STATE.NORMAL.COLD [order 1] : [(flt_HOT <= CD_HOT_COLD)...
          | && (state_Engine == ENGINE_RUNNING)]
      ERROR_STATE.NORMAL.COLD -> ERROR_STATE.NORMAL.NORMAL : [(flt_HOT > (CD_HOT_COLD + CD_TEMPERATURE_HYSTERESIS))...
          | || (state_Engine != ENGINE_RUNNING)]
    state OORL
      state DEBOUNCE
        en:debounceCount = 0;
        du:debounceCount++;
      state NORMAL
        en:state_HOT= OORL;
      (default) -> ERROR_STATE.OORL.DEBOUNCE
      ERROR_STATE.OORL.DEBOUNCE -> ERROR_STATE.OORL.NORMAL : [(debounceCount >= CD_HOT_DEBOUNCE_OORL)...
          | || (state_HOT == OORL)]
    (default) -> NON_FUNCTIONAL
    OORL -> ERROR_STATE.NORMAL [order 1] : [(rm_HOT > CD_HOT_OORL)]
    NON_FUNCTIONAL -> ERROR_STATE.NORMAL : [(state_SensorSupply1 == NORMAL)...
        | && (state_System == SYS_NORMAL)]
    ERROR_STATE.NORMAL -> NON_FUNCTIONAL [order 1] : [(state_SensorSupply1 != NORMAL)...
        | || (state_System != SYS_NORMAL)]
    OORH -> ERROR_STATE.NORMAL [order 1] : [(rm_HOT < CD_HOT_OORH)]
    ERROR_STATE.NORMAL -> OORH [order 2] : [(state_HOT != SHUTDOWN)...
        | && (rm_HOT >= CD_HOT_OORH)]
    ERROR_STATE.NORMAL -> OORL [order 3] : [(state_HOT != SHUTDOWN)...
        | && (rm_HOT <= CD_HOT_OORL)]
    OORH -> NON_FUNCTIONAL [order 2] : [(state_SensorSupply1 != NORMAL)...
        | && (state_HOT != OORH)]
    OORL -> NON_FUNCTIONAL [order 2] : [(state_SensorSupply1 != NORMAL)...
        | && (state_HOT != OORL)]
  state VALUE [parallel]
    settings: executionOrder=1
    state INIT
      en:flt_HOT = 0;
      (junction 68) -> (junction 70) [order 1] : [(rm_HOT < CD_HOT_OORL)...
          | || (rm_HOT > CD_HOT_OORH)]
      (junction 70) -> (junction 71) : {
          | flt_HOT = 0;
          | }
      (junction 71) -> (junction 69)
      (junction 68) -> (junction 69) [order 2] : {
          | flt_HOT = flt_HOT_in;
          | }
      (default) -> (junction 68)
    state NORMAL
      du:flt_HOT = flt_HOT_in;
    (default) -> INIT
    INIT -> VALUE.NORMAL : [(state_System == SYS_NORMAL)]
  data: rm_HOT input uint16; flt_HOT_in input uint16; state_HOT output uint8; state_SensorSupply1 input double; CD_HOT_OORH parameter uint16; CD_HOT_OORL parameter uint16; CD_HOT_DEBOUNCE_OORH parameter uint16; CD_HOT_DEBOUNCE_OORL parameter uint16; CD_HOT_DEBOUNCE_NORMAL parameter uint16; CD_HOT_DEBOUNCE_HIGH parameter uint16; CD_HOT_DEBOUNCE_COLD parameter uint16; CD_HOT_DEBOUNCE_EXTREMELY_HIGH parameter uint16; CD_HOT_DEBOUNCE_SHUTDOWN parameter uint16; CD_HOT_HIGH parameter uint16; CD_HOT_EXTREMELY_HIGH parameter uint16; CD_HOT_COLD parameter uint16; debounceCount local uint16 =0; CD_SHUTDOWN_FUNCTION parameter uint8; CD_TEMPERATURE_HYSTERESIS parameter uint16; COLD parameter uint8 =12; HIGH parameter uint8 =10; NON_FUNCTIONAL parameter uint8 =255; OORH parameter uint8 =21; OORL parameter uint8 =22; SHUTDOWN parameter uint8 =15; NORMAL parameter uint8 =8; EXTREMELY_HIGH parameter uint8 =11; state_System input uint8; SYS_NORMAL parameter uint8; state_Engine input uint8; ENGINE_RUNNING parameter uint8; flt_HOT output uint16
